simulink model "sim_movement"  (R2021b)
settings: Solver=ode23t  StartTime=0.0  StopTime=5  RelTol=1e-3  EnableMultiTasking=on
model workspace (MAT data in the model file):
  B : Simulink.Parameter (value not decoded)
  J : Simulink.Parameter (value not decoded)
  Ka : Simulink.Parameter (value not decoded)
  Km : Simulink.Parameter (value not decoded)
  L : Simulink.Parameter (value not decoded)
  R : Simulink.Parameter (value not decoded)
values from neighbouring files (symbols this model uses):
  X = -.040    (= -0.04)    [coord.m]
  Y = .22    (= 0.22)    [coord.m]
symbols that are objects in the model workspace (value not decoded): B, J, Ka, Km, L, R
undefined symbols (not defined in the file or in its folder): Z
libraries: sm_lib x58, nesl_utility x3, slpidlib x2, fl_lib x2
(part 2 of 2)

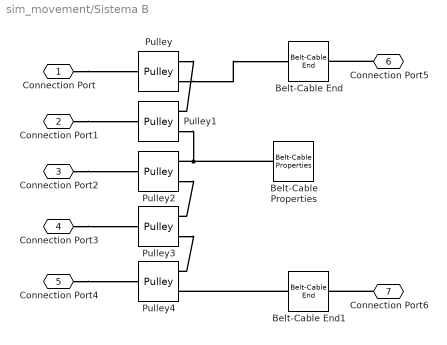
== system sim_movement/Sistema B  ==
  Belt-Cable Properties : sm_lib/Belts and Cables/Belt-Cable Properties  DrumBeltCableAlignment=Unrestricted  GraphicType=PitchLine  GraphicVisPropType=SimpleVisualProperties  GraphicDiffuseColor=[0.5 0.5 0.5]  GraphicSpecularColor=[0.5 0.5 0.5 1.0]  GraphicAmbientColor=[0.15 0.15 0.15 1.0]  GraphicEmissiveColor=[0.0 0.0 0.0 1.0]  GraphicShininess=75  GraphicOpacity=1.0
      settings: SourceProductBaseCode=MS
  Belt-Cable End : sm_lib/Belts and Cables/Belt-Cable End
      settings: SourceProductBaseCode=MS
  Belt-Cable End1 : sm_lib/Belts and Cables/Belt-Cable End
      settings: SourceProductBaseCode=MS
  Pulley{,2..4} (4 alike) : sm_lib/Belts and Cables/Pulley  PitchRadius=3  PitchRadiusUnits=mm  InitialWrapAngleLowerBound=0.0  InitialWrapAngleLowerBoundUnits=deg  SenseWrapAngle=off  SensePulleyAngleA=off  SensePulleyAngleB=off  SenseFleetAngleA=off  SenseFleetAngleB=off
      settings: SourceProductBaseCode=MS
  Pulley1 : sm_lib/Belts and Cables/Pulley  PitchRadius=10  PitchRadiusUnits=mm  InitialWrapAngleLowerBound=0.0  InitialWrapAngleLowerBoundUnits=deg  SenseWrapAngle=off  SensePulleyAngleA=off  SensePulleyAngleB=off  SenseFleetAngleA=off  SenseFleetAngleB=off
      settings: SourceProductBaseCode=MS
  Connection Port : PMIOPort  Side=Left
  Connection Port1 : PMIOPort  Port=2  Side=Left
  Connection Port2 : PMIOPort  Port=3  Side=Left
  Connection Port3 : PMIOPort  Port=4  Side=Left
  Connection Port4 : PMIOPort  Port=5  Side=Left
  Connection Port5 : PMIOPort  Port=6  Side=Left
  Connection Port6 : PMIOPort  Port=7  Side=Left
  connections:
  Connection Port/RConn1 -- Pulley/LConn1
  Connection Port1/RConn1 -- Pulley1/LConn1
  Connection Port2/RConn1 -- Pulley2/LConn1
  Connection Port3/RConn1 -- Pulley3/LConn1
  Connection Port4/RConn1 -- Pulley4/LConn1
  Pulley2/RConn1 -- Pulley1/RConn2 -- Belt-Cable Properties/LConn1
  Pulley2/RConn2 -- Pulley3/RConn1
  Pulley3/RConn2 -- Pulley4/RConn1
  Belt-Cable End1/RConn1 -- Pulley4/RConn2
  Connection Port5/RConn1 -- Belt-Cable End/LConn1
  Connection Port6/RConn1 -- Belt-Cable End1/LConn1
  Pulley/RConn2 -- Belt-Cable End/RConn1
  Pulley/RConn1 -- Pulley1/RConn1
